simulink model "DFPD_SA_MdlIdent"  (R2017a)
settings: Solver=VariableStepAuto  StartTime=0.0  StopTime=150  FixedStep=0.001  EnableMultiTasking=on
PostLoadFcn:
  | , if any(exist('dsrtsu_mdlpostloadfcn', 'file') == [2, 3, 6]), try dsrtsu_mdlpostloadfcn('Execute', bdroot); catch fprintf('Error in PostLoadFcn (dsrtsu_mdlpostloadfcn) for model "%s":\n %s\n', bdroot, lasterr); end, end,
undefined symbols (not defined in the file or in its folder): DFPD_SingleActing, mdlPara, PASL_Models
libraries: PASL_Mechanics x4, PASL_Pneumatics x2, PASL_Components x1, PASL_Tools x1
settings Model: DSRTSU_INTERNAL_RTI_VER=500  DSRTSU_INTERNAL_RTI_TYPE=rti1401  DSRTSU_INTERNAL_RTIFPGA=90  Creator=fbwk  LastModifiedBy=fbwk
settings DataIOCC: LimitDataPoints=on  SaveFormat=Array
settings OptimizationCC: BlockReduction=off  OptimizeBlockIOStorage=off  BufferReuse=off  GlobalBufferReuse=off  ExpressionFolding=off  LocalBlockOutputs=off  LifeSpan=inf
settings DebuggingCC: SolverPrmCheckMsg=warning  SFUnexpectedBacktrackingDiag=warning  SFNoUnconditionalDefaultTransitionDiag=warning  SFExecutionAtInitializationDiag=none
settings HardwareCC: ProdBitPerPointer=32  ProdBitPerSizeT=32  ProdBitPerPtrDiffT=32  ProdLargestAtomicInteger=Integer  ProdEndianess=BigEndian  ProdWordSize=32  ProdHWDeviceType=Custom Processor->Custom  TargetIntDivRoundTo=Zero  TargetEndianess=BigEndian  TargetHWDeviceType=Custom Processor->Custom
settings ModelReferenceCC: PropagateSignalLabelsOutOfModel=off
settings SFSimCC: MATLABDynamicMemAlloc=off
settings RTWCC: SystemTargetFile=rti1005.tlc  MakeCommand=make_rti  TemplateMakefile=rti1005.tmf  Description=dSPACE DS1005 Hardware Platform
settings STFCustomTargetCC: ParMdlRefBuildCompliant=on  MatFileLogging=on  GRTInterface=off  SystemTargetFile=rti1005.tlc
settings GRTTargetCC: TargetLangStandard=C89/C90 (ANSI)  CompOptLevelCompliant=off  ConcurrentExecutionCompliant=off  CombineOutputUpdateFcns=off  CPPClassGenCompliant=off  UseToolchainInfoCompliant=off  ExtModeMexFile=noextcomm
settings ConfigComp: CovMetricSettings=dw  CovHtmlReporting=on  CovSaveCumulativeToWorkspaceVar=on  CovSaveSingleToWorkspaceVar=on  CovExternalEMLEnable=off  CovSFcnEnable=off

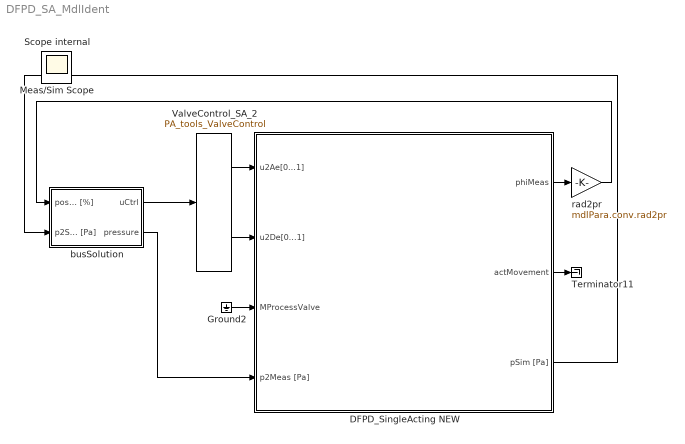
== system DFPD_SA_MdlIdent ==
  DFPD_SingleActing NEW : Subsystem  AncestorBlock=PASL_Models/DFPD_SingleActing  TreatAsAtomicUnit=on  mask(Einfachwirkender DFPD){mdlPara=mdlPara}
      mask prompts: mdlPara "Name of the parameters struct:"
      mask help:
      | Dieses Subsystem beinhaltet das Modell eines
      | einfachwirkenden DFPDs.
      |
      | Zur Initialisierung des Systems kann entweder
      | a) ein vorhandener Parametersatz geladen werden
      | oder
      | b) ein default Datensatz generiert werden.
      | Dabei werden die Daten des DFPD abgefragt
      | und alle aus der Konstruktion bekannten
      | Parameter entsprechend berechnet.
      |
      | !!Bisher ist das Reibungsmodell von Zahnstange
      | und Ritzel mit den Defaultwerten parametriert!!!
      |
      | 2016-03-31, lusc
      mask DialogControl Container4 Prompt: Parameter
      mask DialogControl Control5 Prompt: Parametersatz laden
      mask DialogControl Control5 Callback:
      | %% Modellparameter laden %%%%%%%%%%%%%%%%%%%%%%%%%%%%%%%%%%%%%%%%%%%%%%%%%%
      | 
      | % get mask parameters
      | maskval = get_param(gcb,'MaskValues');
      | structName = maskval{1};
      | 
      | % load parameters
      | assignin('base',structName,...
      | 	aux_loadMdlPara('DFPD')...
      | 	);
      | 
      | % clear section
      | clear maskval structName
      mask DialogControl Control6 Prompt: Parametersatz generieren
      mask DialogControl Control6 Callback:
      | %% Modellparameter laden %%%%%%%%%%%%%%%%%%%%%%%%%%%%%%%%%%%%%%%%%%%%%%%%%%
      | 
      | % get mask parameters
      | maskval = get_param(gcb,'MaskValues');
      | structName = maskval{1};
      | 
      | % load parameters
      | assignin('base',structName,aux_initMdlParaDFPD_SA());
      | 
      | % clear section
      | clear maskval structName
      mask Display:
      | image('DFPD_SingleActing.jpg')
      | 
      | color('black')
      | port_label('input',1,'u2Ae [0...1]')
      | port_label('input',2,'u2De [0...1]')
      | port_label('input',3,'MProcessValve')
      | port_label('input',4,'p2 [Pa] (optional)')
      | 
      | port_label('output',1,'phiMeas [rad]')
      | port_label('output',2,'actMovement')
  Ground2 : Ground
  Terminator11 : Terminator
  ValveControl_SA_2 : PASL_Tools/PA_tools_ValveControl
      settings: SourceProductName=PASL
  busSolution : Subsystem  VariantControl=busVariant
  rad2pr : Gain  Gain=mdlPara.conv.rad2pr
  Meas/Sim Scope : Scope
  Scope internal : Scope
  wires:
  ValveControl_SA_2/2 -> DFPD_SingleActing NEW/2(u2De[0...1])
  Ground2/1 -> DFPD_SingleActing NEW/3("MProcessValve ")
  DFPD_SingleActing NEW/2(actMovement) -> Terminator11/1
  DFPD_SingleActing NEW/1(phiMeas) -> rad2pr/1
  busSolution/2(pressure) -> DFPD_SingleActing NEW/4(p2Meas [Pa])
  ValveControl_SA_2/1 -> DFPD_SingleActing NEW/1(u2Ae[0...1])
  rad2pr/1 -> busSolution/1(posSim [%])
  busSolution/1(uCtrl) -> ValveControl_SA_2/1
  DFPD_SingleActing NEW/3(pSim [Pa]) -> busSolution/2(p2Sim [Pa])

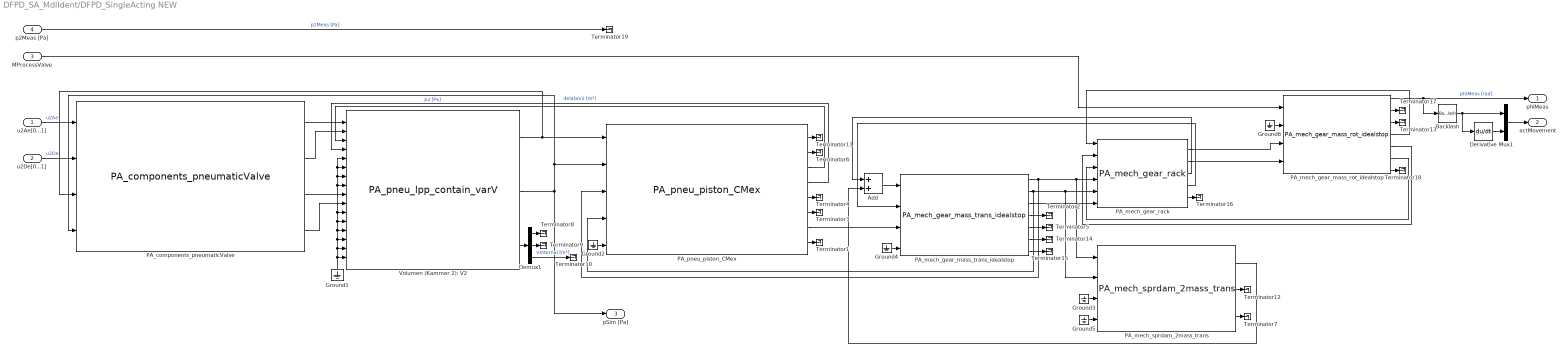
== system DFPD_SA_MdlIdent/DFPD_SingleActing NEW ==
  u2Ae[0...1] : Inport
  u2De[0...1] : Inport  Port=2
  "MProcessValve " : Inport  Port=3
  p2Meas [Pa] : Inport  Port=4
  Add : Sum
  Backlash : Backlash  BacklashWidth=mdlPara.backlash
  Demux1 : Demux  Outputs=3
  Derivative : Derivative
  Ground{1..6} (6 alike) : Ground
  Mux1 : Mux  Inputs=2
  PA_components_pneumaticValve : PASL_Components/PA_components_pneumaticValve  b=mdlPara.b  C=mdlPara.C2  pv=mdlPara.pv  pu=mdlPara.pu  Tu=mdlPara.Tu  R=mdlPara.R  n=mdlPara.n  smoothFact=mdlPara.smoothFac
      settings: SourceProductName=PASL
  PA_mech_gear_mass_rot_idealstop : PASL_Mechanics/Gear Elements/PA_mech_gear_mass_rot_idealstop  Tag=RB_mech_gear_mass_rot_idealstop  phiinit=mdlPara.phi0  phidotinit=mdlPara.phiDot0  J=mdlPara.inertia  drot1=mdlPara.pinionViscFri  drot2=0.0  drot3=0.0  phidotstri=mdlPara.pinionStribeckVel  Mstick=mdlPara.pinionMstick  Mslip=mdlPara.pinionMcoulomb  phimin=mdlPara.phiMin  phimax=mdlPara.phiMax
      settings: SourceProductName=PASL
  PA_mech_gear_mass_trans_idealstop : PASL_Mechanics/Gear Elements/PA_mech_gear_mass_trans_idealstop  Tag=RB_mech_gear_mass_rot_idealstop  xinit=mdlPara.x0  xdotinit=mdlPara.v0  m=mdlPara.mass  dtrans1=mdlPara.viscFriCoeff1  dtrans2=0.0  dtrans3=0.0  xdotstri=mdlPara.stribeckVel  Fstick=mdlPara.Fstick  Fslip=mdlPara.Fcoulomb  xmin=mdlPara.xMin  xmax=mdlPara.xMax
      settings: SourceProductName=PASL
  PA_mech_gear_rack : PASL_Mechanics/Gear Elements/PA_mech_gear_rack  Tag=RB_mech_gear_rack_partrans  r2=mdlPara.pitchRadius  lot=mdlPara.lot  dx0=mdlPara.initRelShift  cgeartrans=mdlPara.gearStiffness  dgeartrans=mdlPara.gearDamp  Fdmax=mdlPara.maxDampForce  eta=mdlPara.eta  etamode=mode 1: robust
      settings: SourceProductName=PASL
  PA_mech_sprdam_2mass_trans : PASL_Mechanics/Spring and Damping Elements/PA_mech_sprdam_2mass_trans  Tag=PA_mech_sprdam_2mass_trans  ctrans=mdlPara.c  dtrans=mdlPara.d  x0=mdlPara.xfZero  lot=mdlPara.transLot
      settings: SourceProductName=PASL
  PA_pneu_piston_CMex : PASL_Pneumatics/Pistons/PA_pneu_piston_CMex  d_out=mdlPara.d2Out  d_in=mdlPara.d2In  p0=mdlPara.pu  x_0=mdlPara.x0
      settings: SourceProductName=PASL
  Terminator{1..19} (19 alike) : Terminator
  Volumen (Kammer 2): V2 : PASL_Pneumatics/Volumes/PA_pneu_lpp_contain_varV  p0=mdlPara.p02  T0=mdlPara.Tu  V0=mdlPara.V02  K=mdlPara.heatExCoeff  A=mdlPara.heatExArea  Tw=mdlPara.Tu  R=mdlPara.R  kappa=mdlPara.n  temp_effects=without temperature effects
      settings: SourceProductName=PASL
  phiMeas : Outport
  actMovement : Outport  Port=2
  pSim [Pa] : Outport  Port=3
  wires:
  Ground3/1 -> PA_mech_sprdam_2mass_trans/3
  Demux1/3 -> Terminator10/1  "VInternal [m³]"
  Demux1/2 -> Terminator9/1
  Demux1/1 -> Terminator8/1
  Volumen (Kammer 2): V2/3 -> Demux1/1
  Derivative/1 -> Mux1/2
  Backlash/1 -> Mux1/1, Derivative/1
  Mux1/1 -> actMovement/1
  Ground1/1 -> Volumen (Kammer 2): V2/16, Volumen (Kammer 2): V2/12, Volumen (Kammer 2): V2/5, Volumen (Kammer 2): V2/6, Volumen (Kammer 2): V2/7, Volumen (Kammer 2): V2/8, Volumen (Kammer 2): V2/11, Volumen (Kammer 2): V2/13, Volumen (Kammer 2): V2/14, Volumen (Kammer 2): V2/15
  "MProcessValve "/1 -> PA_mech_gear_mass_rot_idealstop/1
  PA_mech_gear_mass_rot_idealstop/3 -> Terminator13/1
  PA_mech_gear_mass_rot_idealstop/2 -> Terminator17/1
  PA_mech_gear_mass_rot_idealstop/1 -> phiMeas/1, Backlash/1  "phiMeas [rad]"
  u2De[0...1]/1 -> PA_components_pneumaticValve/2  "u2De"
  u2Ae[0...1]/1 -> PA_components_pneumaticValve/1  "u2Ae"
  PA_pneu_piston_CMex/3 -> Volumen (Kammer 2): V2/3
  PA_pneu_piston_CMex/4 -> Volumen (Kammer 2): V2/4  "delataV2 [m³]"
  PA_pneu_piston_CMex/8 -> Terminator1/1
  Volumen (Kammer 2): V2/2 -> PA_components_pneumaticValve/4, PA_pneu_piston_CMex/2, pSim [Pa]/1  "p2 [Pa]"
  PA_mech_gear_rack/2 -> PA_mech_gear_mass_rot_idealstop/4
  Ground6/1 -> PA_mech_gear_mass_rot_idealstop/2
  PA_mech_gear_mass_rot_idealstop/7 -> Terminator18/1
  Ground4/1 -> PA_mech_gear_mass_trans_idealstop/4
  PA_mech_gear_mass_trans_idealstop/6 -> Terminator14/1
  PA_mech_gear_rack/4 -> PA_mech_gear_mass_trans_idealstop/2
  PA_mech_gear_rack/1 -> PA_mech_gear_mass_rot_idealstop/3
  PA_mech_gear_mass_trans_idealstop/7 -> Terminator15/1
  PA_mech_gear_rack/5 -> Terminator16/1
  PA_mech_gear_mass_rot_idealstop/5 -> PA_mech_gear_rack/2
  PA_mech_gear_mass_rot_idealstop/4 -> PA_mech_gear_rack/1
  PA_mech_gear_mass_rot_idealstop/6 -> PA_mech_gear_rack/3
  PA_mech_gear_mass_trans_idealstop/2 -> PA_mech_sprdam_2mass_trans/2, PA_mech_gear_rack/5, PA_pneu_piston_CMex/4
  Volumen (Kammer 2): V2/1 -> PA_pneu_piston_CMex/1, PA_components_pneumaticValve/3
  PA_pneu_piston_CMex/5 -> Terminator4/1
  PA_pneu_piston_CMex/6 -> Terminator3/1
  Ground5/1 -> PA_mech_sprdam_2mass_trans/4
  PA_mech_sprdam_2mass_trans/3 -> Terminator7/1
  PA_pneu_piston_CMex/2 -> Terminator6/1
  PA_mech_sprdam_2mass_trans/2 -> Terminator12/1
  PA_mech_gear_mass_trans_idealstop/3 -> PA_mech_gear_rack/6
  PA_mech_gear_rack/3 -> Add/1
  Add/1 -> PA_mech_gear_mass_trans_idealstop/1
  Ground2/1 -> PA_pneu_piston_CMex/5
  PA_mech_gear_mass_trans_idealstop/1 -> PA_mech_sprdam_2mass_trans/1, PA_mech_gear_rack/4, PA_pneu_piston_CMex/3
  PA_pneu_piston_CMex/7 -> PA_mech_gear_mass_trans_idealstop/3
  PA_pneu_piston_CMex/1 -> Terminator11/1
  PA_mech_sprdam_2mass_trans/1 -> Add/2
  PA_components_pneumaticValve/1 -> Volumen (Kammer 2): V2/1
  PA_components_pneumaticValve/2 -> Volumen (Kammer 2): V2/2
  PA_components_pneumaticValve/3 -> Volumen (Kammer 2): V2/9
  PA_components_pneumaticValve/4 -> Volumen (Kammer 2): V2/10
  p2Meas [Pa]/1 -> Terminator19/1  "p2Meas [Pa]"
  PA_mech_gear_mass_trans_idealstop/5 -> Terminator5/1
  PA_mech_gear_mass_trans_idealstop/4 -> Terminator2/1

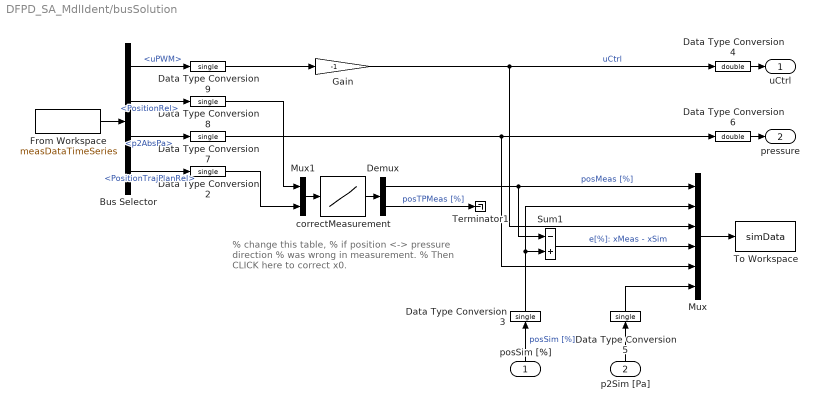
== system DFPD_SA_MdlIdent/busSolution ==
  note: % change this table,
      | % if position <-> pressure direction
      | % was wrong in measurement.
      | % Then CLICK here to correct x0.
  posSim [%] : Inport
  p2Sim [Pa] : Inport  Port=2
  Bus Selector : BusSelector  OutputSignals=uPWM,PositionRel,p2AbsPa,PositionTrajPlanRel
  Data Type Conversion{2..3,5,7..9} (6 alike) : DataTypeConversion  OutDataTypeStr=single
  Data Type Conversion4 : DataTypeConversion  OutDataTypeStr=double
  Data Type Conversion6 : DataTypeConversion  OutDataTypeStr=double
  Demux : Demux  Outputs=2
  From Workspace : FromWorkspace  VariableName=measDataTimeSeries  OutDataTypeStr=Bus: busMeasData  SampleTime=0
  Gain : Gain  Gain=-1
  Mux : Mux  Inputs=6
  Mux1 : Mux  Inputs=2
  Sum1 : Sum  Inputs=-+
  Terminator1 : Terminator
  To Workspace : ToWorkspace  VariableName=simData  SaveFormat=Structure With Time  SampleTime=-1
  correctMeasurement : Lookup_n-D  NumberOfTableDimensions=1  BreakpointsForDimension1=[0,100]  Table=[100,0]  InternalRulePriority=Speed  RndMeth=Simplest  InputSameDT=on
  uCtrl : Outport
  pressure : Outport  Port=2
  wires:
  Data Type Conversion4/1 -> uCtrl/1
  Data Type Conversion3/1 -> Mux/2, Sum1/2
  Demux/1 -> Sum1/1, Mux/1  "posMeas [%]"
  Gain/1 -> Data Type Conversion4/1, Mux/3  "uCtrl"
  Mux/1 -> To Workspace/1
  Sum1/1 -> Mux/4  "e[%]: xMeas - xSim"
  posSim [%]/1 -> Data Type Conversion3/1  "posSim [%]"
  Bus Selector/2 -> Data Type Conversion8/1  "<PositionRel>"
  From Workspace/1 -> Bus Selector/1
  Bus Selector/1 -> Data Type Conversion9/1  "<uPWM>"
  Bus Selector/3 -> Data Type Conversion7/1  "<p2AbsPa>"
  Bus Selector/4 -> Data Type Conversion2/1  "<PositionTrajPlanRel>"
  Demux/2 -> Terminator1/1  "posTPMeas [%]"
  Mux1/1 -> correctMeasurement/1
  correctMeasurement/1 -> Demux/1
  p2Sim [Pa]/1 -> Data Type Conversion5/1
  Data Type Conversion5/1 -> Mux/6
  Data Type Conversion6/1 -> pressure/1
  Data Type Conversion7/1 -> Mux/5, Data Type Conversion6/1
  Data Type Conversion2/1 -> Mux1/2
  Data Type Conversion8/1 -> Mux1/1
  Data Type Conversion9/1 -> Gain/1
